simulink model "pendule_simple2"  (R2016a)
settings: Solver=FixedStepAuto  StartTime=0.0  StopTime=100  FixedStep=0.01  RelTol=1e-3
libraries: simulink x1
settings Model: Creator=nsurbayr  LastModifiedBy=nsurbayr

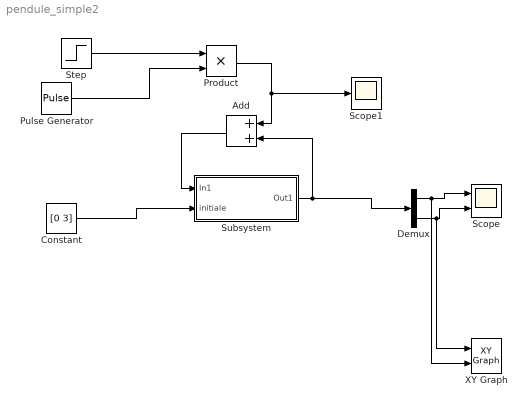
== system pendule_simple2 ==
  Add : Sum
  Constant : Constant  Value=[0 3]
  Demux : Demux  Outputs=2
  Product : Product
  Pulse Generator : DiscretePulseGenerator  PulseType=Time based  Amplitude=[1 0]  Period=10  PulseWidth=10  PhaseDelay=15  VectorParams1D=off
  Scope : Scope  NumInputPorts=2
  Scope1 : Scope
  Step : Step  Time=25  Before=1  After=0  SampleTime=0
  Subsystem : Subsystem
  XY Graph : simulink/Sinks/XY Graph  xmin=-50  xmax=20  ymin=-5  ymax=5  st=-1
  wires:
  Subsystem/1(Out1) -> Add/2, Demux/1
  Constant/1 -> Subsystem/2(initiale)
  Demux/2 -> XY Graph/1, Scope/2
  Demux/1 -> XY Graph/2, Scope/1
  Add/1 -> Subsystem/1(In1)
  Product/1 -> Scope1/1, Add/1
  Step/1 -> Product/1
  Pulse Generator/1 -> Product/2

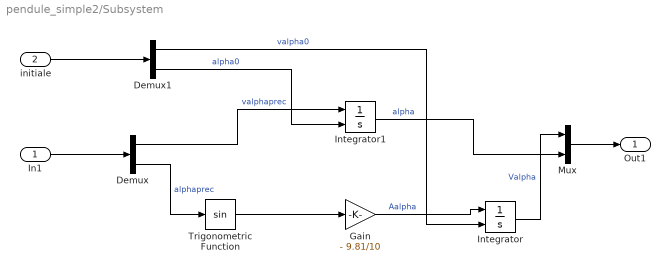
== system pendule_simple2/Subsystem ==
  In1 : Inport
  initiale : Inport  Port=2
  Demux : Demux  Outputs=2
  Demux1 : Demux  Outputs=2
  Gain : Gain  Gain=- 9.81/10
  Integrator : Integrator  InitialConditionSource=external
  Integrator1 : Integrator  InitialConditionSource=external  InitialCondition=pi
  Mux : Mux  Inputs=2
  Trigonometric Function : Trigonometry
  Out1 : Outport
  wires:
  Gain/1 -> Integrator/1  "Aalpha"
  Trigonometric Function/1 -> Gain/1
  In1/1 -> Demux/1
  Demux/2 -> Trigonometric Function/1  "alphaprec"
  Mux/1 -> Out1/1
  Integrator1/1 -> Mux/2  "alpha"
  Integrator/1 -> Mux/1  "Valpha"
  Demux/1 -> Integrator1/1  "valphaprec"
  initiale/1 -> Demux1/1
  Demux1/2 -> Integrator1/2  "alpha0"
  Demux1/1 -> Integrator/2  "valpha0"
